simulink model "Delete"  (R2020a)
settings: Solver=VariableStepAuto  StartTime=0.0  StopTime=10.0  RelTol=1e-3
undefined symbols (not defined in the file): d1, d2, k1, k2, m1, m2
settings Model: Creator=wxcli  LastModifiedBy=wxcli

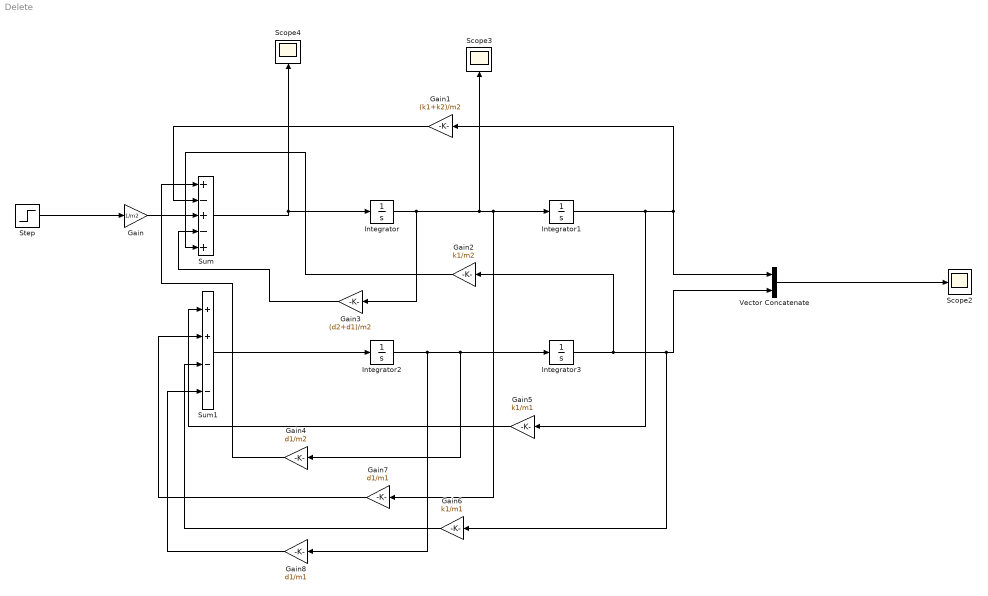
== system Delete ==
  Gain : Gain  Gain=1/m2
  Gain1 : Gain  Gain=(k1+k2)/m2
  Gain2 : Gain  Gain=k1/m2
  Gain3 : Gain  Gain=(d2+d1)/m2
  Gain4 : Gain  Gain=d1/m2
  Gain5 : Gain  Gain=k1/m1
  Gain6 : Gain  Gain=k1/m1
  Gain7 : Gain  Gain=d1/m1
  Gain8 : Gain  Gain=d1/m1
  Integrator{,1..3} (4 alike) : Integrator
  Scope2 : Scope
  Scope3 : Scope
  Scope4 : Scope
  Step : Step  SampleTime=0
  Sum : Sum  Inputs=+-+-+
  Sum1 : Sum  Inputs=++--
  Vector Concatenate : Concatenate
  wires:
  Gain4/1 -> Sum/1
  Gain1/1 -> Sum/2
  Sum/1 -> Scope4/1, Integrator/1
  Vector Concatenate/1 -> Scope2/1
  Integrator/1 -> Gain3/1, Scope3/1, Gain7/1, Integrator1/1
  Gain2/1 -> Sum/5
  Gain8/1 -> Sum1/4
  Gain3/1 -> Sum/4
  Gain7/1 -> Sum1/2
  Gain/1 -> Sum/3
  Integrator3/1 -> Gain2/1, Gain6/1, Vector Concatenate/2
  Integrator1/1 -> Gain5/1, Vector Concatenate/1, Gain1/1
  Gain6/1 -> Sum1/3
  Gain5/1 -> Sum1/1
  Integrator2/1 -> Gain8/1, Gain4/1, Integrator3/1
  Sum1/1 -> Integrator2/1
  Step/1 -> Gain/1
